simulink model "DAB_batteryload"  (R2024b)
settings: Solver=ode15s  StartTime=0.0  StopTime=1  RelTol=1e-3
undefined symbols (not defined in the file): Acid, Lead, sigbuilder_block
libraries: spsIGBTDiodeLib x8, spsVoltageMeasurementLib x5, spsSeriesRLCBranchLib x4, simulink x3, spsCurrentMeasurementLib x3, spsBatteryLib x2, spsMeanLib x2, spsLinearTransformerLib x1, spspowerguiLib x1
settings Model: Creator=shiekhsoliha  LastModifiedBy=sheikhsoliha
settings SolverCC: AlgebraicLoopSolver=TrustRegion
settings DataIOCC: ReturnWorkspaceOutputs=off
settings OptimizationCC: ReuseModelBlockBuffer=off
settings DebuggingCC: UnconnectedInputMsg=warning  UnconnectedOutputMsg=warning  UnconnectedLineMsg=warning  ArithmeticOperatorsInVariantConditions=warning
settings ModelReferenceCC: EnableRefExpFcnMdlSchedulingChecks=on
settings SFSimCC: SimUseLocalCustomCode=off  CustomCodeUndefinedFunction=UseInterfaceOnly
settings RTWCC: RTWUseLocalCustomCode=off  GPUComputeCapability=3.5

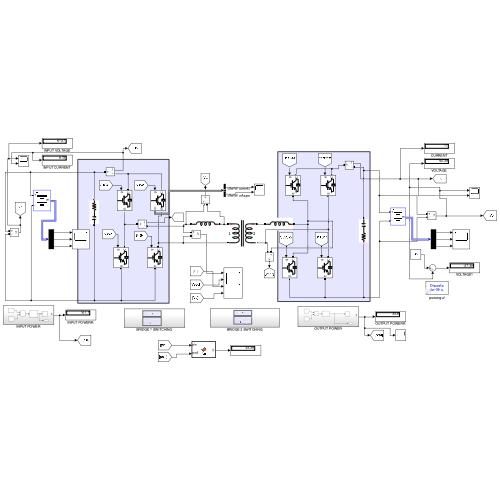
[thumbnail: Simulink's stored preview of the top-level diagram]
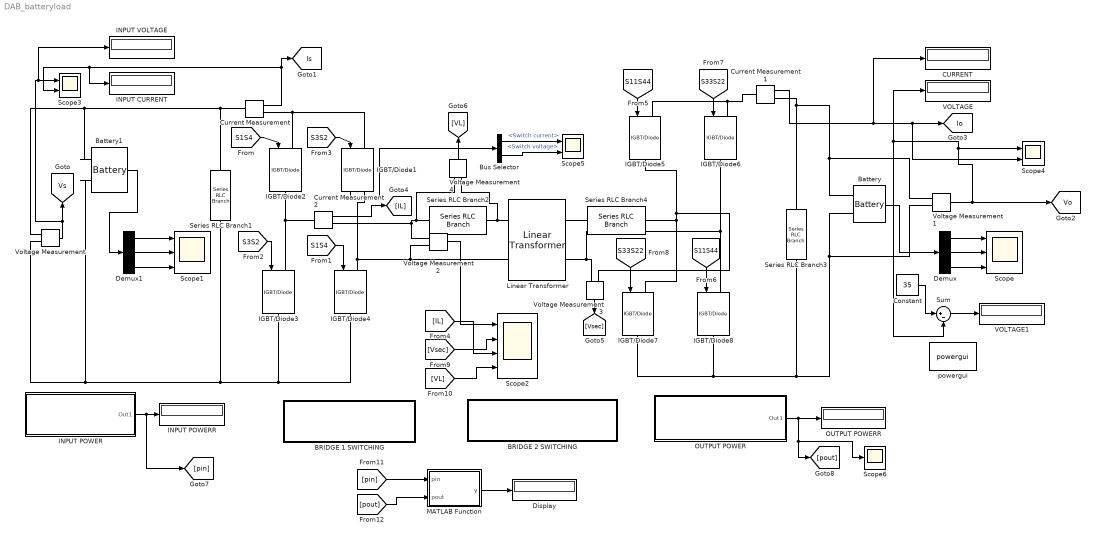
== system DAB_batteryload ==
  BRIDGE 1 SWITCHING : Subsystem
  BRIDGE 2 SWITCHING : Subsystem
  Battery : spsBatteryLib/Battery  BatType=Lead-Acid  NomV=30.5  NomQ=1.5  SOC=90  Batt_Tr=.001  PresetModel=on  MaxQ=1.5625  MinV=22.875  FullV=33.2089  Dis_rate=0.3  R=0.20333  Normal_OP=0.46542  expZone="[31.0518        0.005]"
      settings: LibrarySourceBlock=electricdrivelib/Extra Sources/Battery
  Battery1 : spsBatteryLib/Battery  BatType=Lead-Acid  NomV=300  NomQ=1.5  SOC=90  Batt_Tr=.001  PresetModel=on  MaxQ=1.5625  MinV=225  FullV=326.6447  Dis_rate=0.3  R=2  Normal_OP=0.46542  expZone="[305.4276         0.005]"
      settings: LibrarySourceBlock=electricdrivelib/Extra Sources/Battery
  Bus Selector : BusSelector  OutputSignals=Switch current,Switch voltage
  CURRENT : Display
  Constant : Constant  Value=35
  Current Measurement : spsCurrentMeasurementLib/Current Measurement  PhasorSimulation=off  OutputType=Complex  PSBequivalent=0
  Current Measurement1 : spsCurrentMeasurementLib/Current Measurement  PhasorSimulation=off  OutputType=Complex  PSBequivalent=0
  Current Measurement2 : spsCurrentMeasurementLib/Current Measurement  PhasorSimulation=off  OutputType=Complex  PSBequivalent=0
  Demux : Demux  Outputs=3
  Demux1 : Demux  Outputs=3
  Display : Display
  IGBT/Diode1 : spsIGBTDiodeLib/IGBT//Diode  Ron=1e-3  Rs=1e5  Cs=inf  Measurements=on
  IGBT/Diode{2..8} (7 alike) : spsIGBTDiodeLib/IGBT//Diode  Ron=1e-3  Rs=1e5  Cs=inf  Measurements=off
  INPUT CURRENT : Display
  INPUT POWER : Subsystem
  INPUT POWERR : Display
  INPUT VOLTAGE : Display
  Linear Transformer : spsLinearTransformerLib/Linear Transformer  UNITS=pu  NominalPower=[ 2000 20000 ]  winding1="[ 300 0.017  0.0016 ]"  winding2=[ 100 0.017 .0030 ]  ThreeWindings=off  winding3=[ 315e3 0.002 0.08 ]  RmLm=[ 500 500 ]  Measurements=None  DataType=off
  MATLAB Function : MATLAB Function  TreatAsAtomicUnit=on
  OUTPUT POWER : Subsystem
  OUTPUT POWERR : Display
  Scope : Scope  NumInputPorts=3
  Scope1 : Scope  NumInputPorts=3
  Scope2 : Scope  NumInputPorts=4
  Scope3 : Scope  NumInputPorts=2
  Scope4 : Scope  NumInputPorts=2
  Scope5 : Scope  NumInputPorts=2
  Scope6 : Scope
  Series RLC Branch1 : spsSeriesRLCBranchLib/Series RLC Branch  LConnTagsString=__new0  RConnTagsString=__new0  BranchType=RC  Resistance=.001  Inductance=1e-3  SetiL0=off  InitialCurrent=0  Capacitance=300e-6  Setx0=off  InitialVoltage=0  Measurements=None
  Series RLC Branch2 : spsSeriesRLCBranchLib/Series RLC Branch  LConnTagsString=__new0  RConnTagsString=__new0  BranchType=L  Resistance=.001  Inductance=45e-5  SetiL0=off  InitialCurrent=0  Capacitance=300e-6  Setx0=off  InitialVoltage=0  Measurements=None
  Series RLC Branch3 : spsSeriesRLCBranchLib/Series RLC Branch  LConnTagsString=__new0  RConnTagsString=__new0  BranchType=RC  Resistance=0.001  Inductance=1e-3  SetiL0=off  InitialCurrent=0  Capacitance=4500e-6  Setx0=off  InitialVoltage=0  Measurements=None
  Series RLC Branch4 : spsSeriesRLCBranchLib/Series RLC Branch  LConnTagsString=__new0  RConnTagsString=__new0  BranchType=L  Resistance=.001  Inductance=45e-5  SetiL0=off  InitialCurrent=0  Capacitance=300e-6  Setx0=off  InitialVoltage=0  Measurements=None
  Sum : Sum  Inputs=|+-
  VOLTAGE : Display
  VOLTAGE1 : Display
  Voltage Measurement{,1..4} (5 alike) : spsVoltageMeasurementLib/Voltage Measurement  PhasorSimulation=off  OutputType=Complex  PSBequivalent=0
  powergui : spspowerguiLib/powergui  Priority=1  SimulationMode=Discrete  SampleTime=10e-7  frequency=60  Iterations=50  frequencyindice=0  Pbase=100e6  ErrMax=1e-4  UnitsV=kV  UnitsW=MW  buscounter=0  FunctionMessages=off  echomessages=off  EnableUseOfTLC=off  CurrentSourceSwitches=off  DisableSnubberDevices=off  DisableRonSwitches=off  DisableVfSwitches=off  DisplayEquations=off  AutomaticDiscreteSolvers=off  SolverType=Tustin/Backward Euler (TBE)  Interpol=off  ExternalGateDelay=off  methode=off  Ts=100  x0status=blocks  SPID=off  SwTol=0  HookPort=off  NonlinearTolerance=1e-4  nMaxIteration=100  ContinueOnMaxIteration=off  RestoreLinks=warning  ResistiveCurrentMeasurement=off  Frange=[0:2:500]  Ylog=off  Xlog=on  ShowGrid=off  save=off  variable=ZData  structure=0  ZoomFFT=off  StartTime=0.0  cycles=1  DisplayStyle=1  fundamental=60  FreqAxis=off  MaxFrequency=1000  frequencyindicesteady=1  RmsSteady=1  display=off
  tag scope: Io=global, Is=global, Vo=global, Vs=global
  wires:
  Voltage Measurement/1 -> INPUT VOLTAGE/1, Scope3/1, [Vs]
  Current Measurement/1 -> INPUT CURRENT/1, Scope3/2, [Is]
  [S1S4] -> IGBT/Diode2/1
  [S1S4] -> IGBT/Diode4/1
  [S3S2] -> IGBT/Diode3/1
  [S3S2] -> IGBT/Diode1/1
  [S11S44] -> IGBT/Diode5/1
  [S11S44] -> IGBT/Diode8/1
  [S33S22] -> IGBT/Diode6/1
  [S33S22] -> IGBT/Diode7/1
  Battery/1 -> Demux/1
  Demux/1 -> Scope/1
  Demux/2 -> Scope/2
  Demux/3 -> Scope/3
  Demux1/3 -> Scope1/3
  Demux1/1 -> Scope1/1
  Demux1/2 -> Scope1/2
  Battery1/1 -> Demux1/1
  Current Measurement1/1 -> CURRENT/1, Scope4/2, [Io]
  Current Measurement2/1 -> [IL]
  Voltage Measurement3/1 -> [Vsec]
  Voltage Measurement4/1 -> [VL]
  [Vsec] -> Scope2/2
  Voltage Measurement2/1 -> Scope2/1
  [IL] -> Scope2/3
  [VL] -> Scope2/4
  INPUT POWER/1(Out1) -> [pin], INPUT POWERR/1
  OUTPUT POWER/1(Out1) -> [pout], Scope6/1, OUTPUT POWERR/1
  Voltage Measurement1/1 -> [Vo], VOLTAGE/1, Sum/2, Scope4/1
  Sum/1 -> VOLTAGE1/1
  Constant/1 -> Sum/1
  IGBT/Diode1/1 -> Bus Selector/1
  Bus Selector/1 -> Scope5/1  "<Switch current>"
  Bus Selector/2 -> Scope5/2  "<Switch voltage>"
  [pin] -> MATLAB Function/1(pin)
  [pout] -> MATLAB Function/2(pout)
  MATLAB Function/1(y) -> Display/1
  connections:
  IGBT/Diode3/LConn1 -- IGBT/Diode2/RConn1 -- Current Measurement2/LConn1
  IGBT/Diode1/RConn1 -- Linear Transformer/LConn2 -- Voltage Measurement2/LConn2 -- IGBT/Diode4/LConn1
  IGBT/Diode1/LConn1 -- Current Measurement/RConn1 -- IGBT/Diode2/LConn1
  Series RLC Branch1/RConn1 -- Battery1/LConn2 -- Voltage Measurement/LConn2 -- IGBT/Diode3/RConn1 -- IGBT/Diode4/RConn1
  IGBT/Diode8/LConn1 -- Linear Transformer/RConn2 -- Voltage Measurement3/LConn2 -- IGBT/Diode6/RConn1
  IGBT/Diode5/RConn1 -- Series RLC Branch4/LConn1 -- IGBT/Diode7/LConn1 -- Voltage Measurement3/LConn1
  IGBT/Diode5/LConn1 -- Current Measurement1/LConn1 -- IGBT/Diode6/LConn1
  IGBT/Diode7/RConn1 -- Series RLC Branch3/LConn1 -- Voltage Measurement1/LConn2 -- Battery/LConn2 -- IGBT/Diode8/RConn1
  Battery1/LConn1 -- Voltage Measurement/LConn1 -- Current Measurement/LConn1 -- Series RLC Branch1/LConn1
  Battery/LConn1 -- Voltage Measurement1/LConn1 -- Current Measurement1/RConn1 -- Series RLC Branch3/RConn1
  Current Measurement2/RConn1 -- Voltage Measurement4/LConn1 -- Series RLC Branch2/RConn1 -- Voltage Measurement2/LConn1
  Series RLC Branch2/LConn1 -- Voltage Measurement4/LConn2 -- Linear Transformer/LConn1
  Linear Transformer/RConn1 -- Series RLC Branch4/RConn1

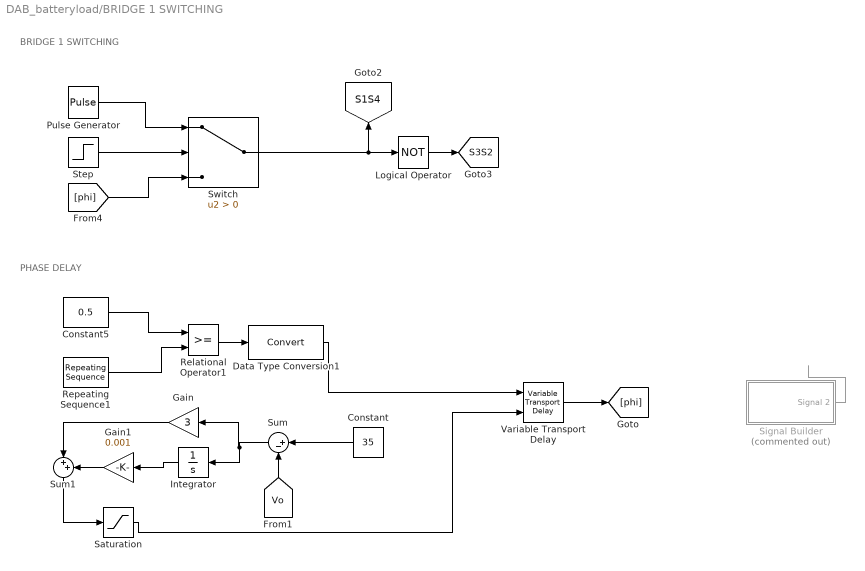
== system DAB_batteryload/BRIDGE 1 SWITCHING ==
  note: PHASE DELAY
  note: BRIDGE 1 SWITCHING
  Constant : Constant  Value=35
  Constant5 : Constant  Value=0.5
  Data Type Conversion1 : DataTypeConversion  SaturateOnIntegerOverflow=off  RndMeth=Floor
  Gain : Gain  Gain=3
  Gain1 : Gain  Gain=0.001
  Integrator : Integrator
  Logical Operator : Logic  Operator=NOT  IconShape=distinctive  AllPortsSameDT=off  OutDataTypeStr=boolean
  Pulse Generator : DiscretePulseGenerator  PulseType=Time based  Period=0.00005  PulseWidth=50
  Relational Operator1 : RelationalOperator  OutDataTypeStr=boolean  InputSameDT=off
  Repeating Sequence1 : simulink/Sources/Repeating Sequence  rep_seq_t=[0 1/20000]  rep_seq_y=[0 1]
  Saturation : Saturate  UpperLimit=35  LowerLimit=-35
  Signal Builder : Subsystem  Tag=STV Subsys  Commented=on  LoadFcn=sigbuilder_block('load');  StartFcn=sigbuilder_block('start');  StopFcn=sigbuilder_block('stop');  ClipboardFcn=sigbuilder_block('clipboard');  mask(Sigbuilder block){tuvar=[0:10]}
      mask help: Simulink:masks:SigbuilderBlock_MD
      mask init:
      | if ~strcmp(get_param(bdroot(gcbh),'SimulationStatus'),'stopped') tuvar = sigbuilder_block('maskInit'); end
      settings: CopyFcn=sigbuilder_block('copy');  DeleteFcn=sigbuilder_block('delete');  ModelCloseFcn=sigbuilder_block('modelClose');  PreSaveFcn=sigbuilder_block('preSave');  PauseFcn=sigbuilder_block('pause');  ContinueFcn=sigbuilder_block('continue');  NameChangeFcn=sigbuilder_block('namechange');  OpenFcn=sigbuilder_block('open',[437.6 199.2 550.4 400 ]);  CloseFcn=sigbuilder_block('close');
      mask Display: plot(0, 0, 100, 100,[2, 2, 32, 32, 2], [68, 8, 8, 68, 68],[32, 2], [38, 38], [32, 19, 2],[53, 60, 44], [32, 17, 17, 2],[16, 16, 31, 31]);txt = getActiveGroup(gcbh);text(2, 100, txt,'verticalAlignment', 'top');
  Step : Step  Time=0.17  Before=.1  After=-.1  SampleTime=0
  Sum : Sum  Inputs=|+-
  Sum1 : Sum  Inputs=|++
  Switch : Switch  Criteria=u2 > Threshold  SaturateOnIntegerOverflow=off  InputSameDT=off
  Variable Transport Delay : VariableTransportDelay  VariableDelayType=Variable transport delay  MaximumDelay=0.0000002125
  tag scope: S1S4=global, S3S2=global
  wires:
  [phi] -> Switch/3
  Step/1 -> Switch/2
  Switch/1 -> [S1S4], Logical Operator/1
  Logical Operator/1 -> [S3S2]
  Pulse Generator/1 -> Switch/1
  [Vo] -> Sum/2
  Gain/1 -> Sum1/1
  Data Type Conversion1/1 -> Variable Transport Delay/1
  Relational Operator1/1 -> Data Type Conversion1/1
  Constant/1 -> Sum/1
  Saturation/1 -> Variable Transport Delay/2
  Constant5/1 -> Relational Operator1/1
  Gain1/1 -> Sum1/2
  Sum/1 -> Integrator/1, Gain/1
  Integrator/1 -> Gain1/1
  Repeating Sequence1/1 -> Relational Operator1/2
  Sum1/1 -> Saturation/1
  Variable Transport Delay/1 -> [phi]
  Signal Builder/1(Signal 2) -> ?

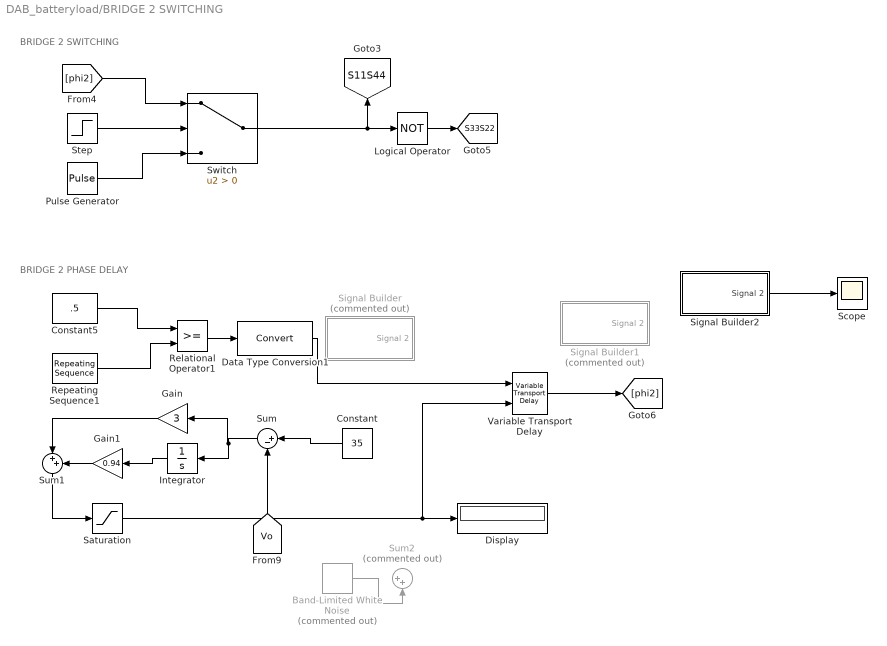
== system DAB_batteryload/BRIDGE 2 SWITCHING ==
  note: BRIDGE 2 PHASE DELAY
  note: BRIDGE 2 SWITCHING
  Band-Limited White Noise : simulink/Sources/Band-Limited White Noise  Commented=on  Cov=[0.1]  Ts=0.1  seed=[23341]
  Constant : Constant  Value=35
  Constant5 : Constant  Value=.5
  Data Type Conversion1 : DataTypeConversion  SaturateOnIntegerOverflow=off  RndMeth=Floor
  Display : Display
  Gain : Gain  Gain=3
  Gain1 : Gain  Gain=0.94
  Integrator : Integrator
  Logical Operator : Logic  Operator=NOT  IconShape=distinctive  AllPortsSameDT=off  OutDataTypeStr=boolean
  Pulse Generator : DiscretePulseGenerator  PulseType=Time based  Period=0.00005  PulseWidth=50
  Relational Operator1 : RelationalOperator  OutDataTypeStr=boolean  InputSameDT=off
  Repeating Sequence1 : simulink/Sources/Repeating Sequence  rep_seq_t=[0 1/20000]  rep_seq_y=[0 1]
  Saturation : Saturate  UpperLimit=35  LowerLimit=-35
  Scope : Scope
  Signal Builder : Subsystem  Tag=STV Subsys  Commented=on  LoadFcn=sigbuilder_block('load');  StartFcn=sigbuilder_block('start');  StopFcn=sigbuilder_block('stop');  ClipboardFcn=sigbuilder_block('clipboard');  mask(Sigbuilder block){tuvar=[0:10]}
      mask help: Simulink:masks:SigbuilderBlock_MD
      mask init:
      | if ~strcmp(get_param(bdroot(gcbh),'SimulationStatus'),'stopped') tuvar = sigbuilder_block('maskInit'); end
      settings: CopyFcn=sigbuilder_block('copy');  DeleteFcn=sigbuilder_block('delete');  ModelCloseFcn=sigbuilder_block('modelClose');  PreSaveFcn=sigbuilder_block('preSave');  PauseFcn=sigbuilder_block('pause');  ContinueFcn=sigbuilder_block('continue');  NameChangeFcn=sigbuilder_block('namechange');  OpenFcn=sigbuilder_block('open',[437.6 199.2 550.4 400 ]);  CloseFcn=sigbuilder_block('close');
      mask Display: plot(0, 0, 100, 100,[2, 2, 32, 32, 2], [68, 8, 8, 68, 68],[32, 2], [38, 38], [32, 19, 2],[53, 60, 44], [32, 17, 17, 2],[16, 16, 31, 31]);txt = getActiveGroup(gcbh);text(2, 100, txt,'verticalAlignment', 'top');
  Signal Builder1 : Subsystem  Tag=STV Subsys  Commented=on  LoadFcn=sigbuilder_block('load');  StartFcn=sigbuilder_block('start');  StopFcn=sigbuilder_block('stop');  ClipboardFcn=sigbuilder_block('clipboard');  mask(Sigbuilder block){tuvar=[0:10]}
      mask help: Simulink:masks:SigbuilderBlock_MD
      mask init:
      | if ~strcmp(get_param(bdroot(gcbh),'SimulationStatus'),'stopped') tuvar = sigbuilder_block('maskInit'); end
      settings: CopyFcn=sigbuilder_block('copy');  DeleteFcn=sigbuilder_block('delete');  ModelCloseFcn=sigbuilder_block('modelClose');  PreSaveFcn=sigbuilder_block('preSave');  PauseFcn=sigbuilder_block('pause');  ContinueFcn=sigbuilder_block('continue');  NameChangeFcn=sigbuilder_block('namechange');  OpenFcn=sigbuilder_block('open',[437.6 199.2 550.4 400 ]);  CloseFcn=sigbuilder_block('close');
      mask Display: plot(0, 0, 100, 100,[2, 2, 32, 32, 2], [68, 8, 8, 68, 68],[32, 2], [38, 38], [32, 19, 2],[53, 60, 44], [32, 17, 17, 2],[16, 16, 31, 31]);txt = getActiveGroup(gcbh);text(2, 100, txt,'verticalAlignment', 'top');
  Signal Builder2 : Subsystem  Tag=STV Subsys  LoadFcn=sigbuilder_block('load');  StartFcn=sigbuilder_block('start');  StopFcn=sigbuilder_block('stop');  ClipboardFcn=sigbuilder_block('clipboard');  mask(Sigbuilder block){tuvar=[0:10]}
      mask help: Simulink:masks:SigbuilderBlock_MD
      mask init:
      | if ~strcmp(get_param(bdroot(gcbh),'SimulationStatus'),'stopped') tuvar = sigbuilder_block('maskInit'); end
      settings: CopyFcn=sigbuilder_block('copy');  DeleteFcn=sigbuilder_block('delete');  ModelCloseFcn=sigbuilder_block('modelClose');  PreSaveFcn=sigbuilder_block('preSave');  PauseFcn=sigbuilder_block('pause');  ContinueFcn=sigbuilder_block('continue');  NameChangeFcn=sigbuilder_block('namechange');  OpenFcn=sigbuilder_block('open',[437.6 199.2 550.4 400 ]);  CloseFcn=sigbuilder_block('close');
      mask Display: plot(0, 0, 100, 100,[2, 2, 32, 32, 2], [68, 8, 8, 68, 68],[32, 2], [38, 38], [32, 19, 2],[53, 60, 44], [32, 17, 17, 2],[16, 16, 31, 31]);txt = getActiveGroup(gcbh);text(2, 100, txt,'verticalAlignment', 'top');
  Step : Step  Time=0.17  Before=.1  After=-.1  SampleTime=0
  Sum : Sum  Inputs=|+-
  Sum1 : Sum  Inputs=|++
  Sum2 : Sum  Commented=on  Inputs=|++
  Switch : Switch  Criteria=u2 > Threshold  SaturateOnIntegerOverflow=off  InputSameDT=off
  Variable Transport Delay : VariableTransportDelay  VariableDelayType=Variable transport delay  MaximumDelay=0.00000075
  tag scope: S11S44=global, S33S22=global
  wires:
  Sum/1 -> Integrator/1, Gain/1
  Integrator/1 -> Gain1/1
  Gain1/1 -> Sum1/2
  Constant5/1 -> Relational Operator1/1
  Pulse Generator/1 -> Switch/3
  Sum1/1 -> Saturation/1
  Logical Operator/1 -> [S33S22]
  Step/1 -> Switch/2
  Variable Transport Delay/1 -> [phi2]
  Switch/1 -> [S11S44], Logical Operator/1
  Data Type Conversion1/1 -> Variable Transport Delay/1
  Relational Operator1/1 -> Data Type Conversion1/1
  Constant/1 -> Sum/1
  Saturation/1 -> Display/1, Variable Transport Delay/2
  Gain/1 -> Sum1/1
  Repeating Sequence1/1 -> Relational Operator1/2
  [Vo] -> Sum/2
  [phi2] -> Switch/1
  Band-Limited White Noise/1 -> Sum2/2
  Signal Builder2/1(Signal 2) -> Scope/1

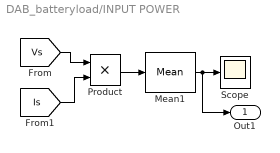
== system DAB_batteryload/INPUT POWER ==
  Mean1 : spsMeanLib/Mean  Freq=60  Vinit=0  Ts=0
  Product : Product
  Scope : Scope
  Out1 : Outport  VectorParamsAs1DForOutWhenUnconnected=off
  wires:
  [Is] -> Product/2
  [Vs] -> Product/1
  Product/1 -> Mean1/1
  Mean1/1 -> Out1/1, Scope/1

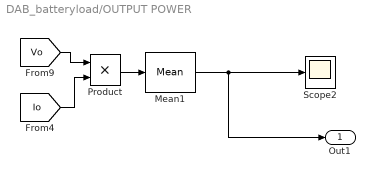
== system DAB_batteryload/OUTPUT POWER ==
  Mean1 : spsMeanLib/Mean  Freq=60  Vinit=0  Ts=0
  Product : Product
  Scope2 : Scope
  Out1 : Outport  VectorParamsAs1DForOutWhenUnconnected=off
  wires:
  [Io] -> Product/2
  Mean1/1 -> Out1/1, Scope2/1
  Product/1 -> Mean1/1
  [Vo] -> Product/1

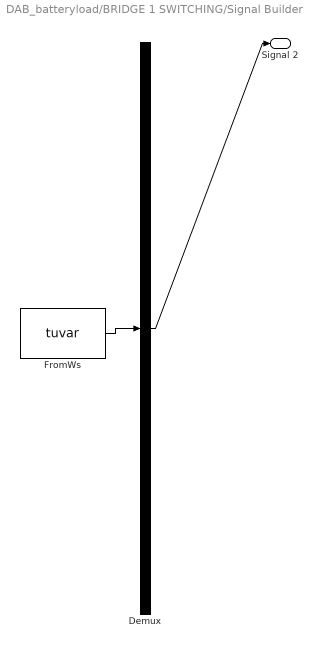
== system DAB_batteryload/BRIDGE 1 SWITCHING/Signal Builder ==
  Demux : Demux  Tag=STV Demux  Outputs=1
      settings: DisplayOption=none
  FromWs : FromWorkspace  Tag=STV FromWs  VariableName=tuvar
      SigBuilderData=|
      | common.afterFinalStr = 'Extrapolate'
      | common.sampleTime = 0
      | dataSet.timeRange = [0 10]
      | dataSet.name = 'Group 1'
      | sbobj.Groups.Name = 'Group 1'
      | sbobj.Groups.Signals.Name = 'Signal 2'
      | sbobj.Groups.Signals.XData = [0 0.1 0.2 0.3 0.4 0.5 0.5 0.6 0.7 0.8 0.9 10]
      | sbobj.Groups.Signals.YData = [35 35 35 35 35 35 25 25 25 25 25 30]
  Signal 2 : Outport  Tag=STV Outport  VectorParamsAs1DForOutWhenUnconnected=off
  wires:
  FromWs/1 -> Demux/1
  Demux/1 -> Signal 2/1

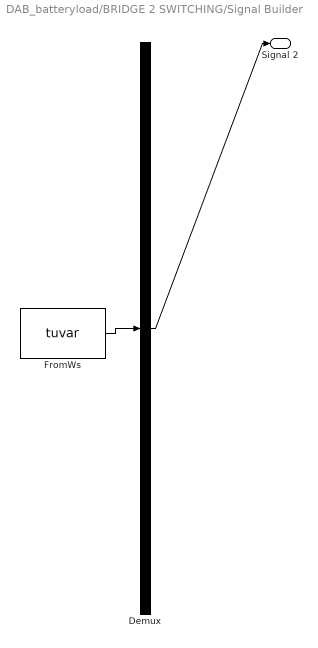
== system DAB_batteryload/BRIDGE 2 SWITCHING/Signal Builder ==
  Demux : Demux  Tag=STV Demux  Outputs=1
      settings: DisplayOption=none
  FromWs : FromWorkspace  Tag=STV FromWs  VariableName=tuvar
      SigBuilderData=|
      | common.afterFinalStr = 'Extrapolate'
      | common.sampleTime = 0
      | dataSet.timeRange = [0 10]
      | dataSet.name = 'Group 1'
      | sbobj.Groups.Name = 'Group 1'
      | sbobj.Groups.Signals.Name = 'Signal 2'
      | sbobj.Groups.Signals.XData = [0 0.1 0.2 0.3 0.4 0.5 0.5 0.6 0.7 0.8 0.9 10]
      | sbobj.Groups.Signals.YData = [35 35 35 35 35 35 25 25 25 25 25 30]
  Signal 2 : Outport  Tag=STV Outport  VectorParamsAs1DForOutWhenUnconnected=off
  wires:
  FromWs/1 -> Demux/1
  Demux/1 -> Signal 2/1

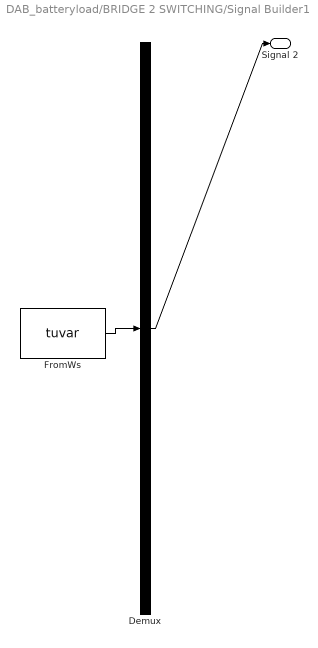
== system DAB_batteryload/BRIDGE 2 SWITCHING/Signal Builder1 ==
  Demux : Demux  Tag=STV Demux  Outputs=1
      settings: DisplayOption=none
  FromWs : FromWorkspace  Tag=STV FromWs  VariableName=tuvar
      SigBuilderData=|
      | common.afterFinalStr = 'Extrapolate'
      | common.sampleTime = 0
      | dataSet.timeRange = [0 10]
      | dataSet.name = 'Group 1'
      | sbobj.Groups.Name = 'Group 1'
      | sbobj.Groups.Signals.Name = 'Signal 2'
      | sbobj.Groups.Signals.XData = [0 0.1 0.2 0.3 0.4 0.5 0.5 0.6 0.7 0.8 0.9 10]
      | sbobj.Groups.Signals.YData = [35 35 35 35 35 35 25 25 25 25 25 30]
  Signal 2 : Outport  Tag=STV Outport  VectorParamsAs1DForOutWhenUnconnected=off
  wires:
  FromWs/1 -> Demux/1
  Demux/1 -> Signal 2/1

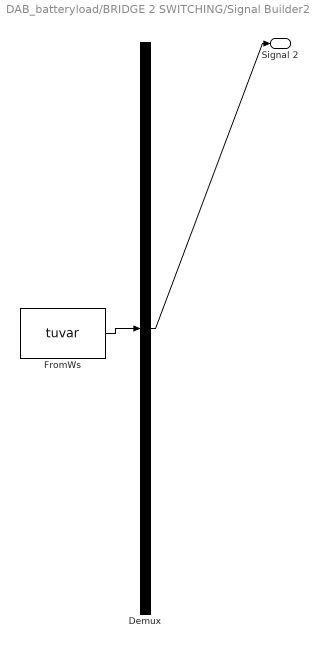
== system DAB_batteryload/BRIDGE 2 SWITCHING/Signal Builder2 ==
  Demux : Demux  Tag=STV Demux  Outputs=1
      settings: DisplayOption=none
  FromWs : FromWorkspace  Tag=STV FromWs  VariableName=tuvar
      SigBuilderData=|
      | common.afterFinalStr = 'Extrapolate'
      | common.sampleTime = 0
      | dataSet.timeRange = [0 10]
      | dataSet.name = 'Group 1'
      | sbobj.Groups.Name = 'Group 1'
      | sbobj.Groups.Signals.Name = 'Signal 2'
      | sbobj.Groups.Signals.XData = [0 0.1 0.2 0.3 0.4 0.5 0.5 0.6 0.7 0.8 0.9 10]
      | sbobj.Groups.Signals.YData = [393 393 393 393 393 393 350 350 350 350 350 350]
  Signal 2 : Outport  Tag=STV Outport  VectorParamsAs1DForOutWhenUnconnected=off
  wires:
  FromWs/1 -> Demux/1
  Demux/1 -> Signal 2/1

== matlab function DAB_batteryload/MATLAB Function ==
  data: pin input; y output; pout input
function y = fcn(pin,pout)
y=(pout/pin)*100;
